simulink model "coursework2model1"  (R2024b)
settings: Solver=VariableStepAuto  StartTime=0.0  StopTime=T  RelTol=1e-3
undefined symbols (not defined in the file): K, x0
settings Model: Creator=user  LastModifiedBy=Oteng_fy0f5z9
settings RTWCC: GPUComputeCapability=3.5

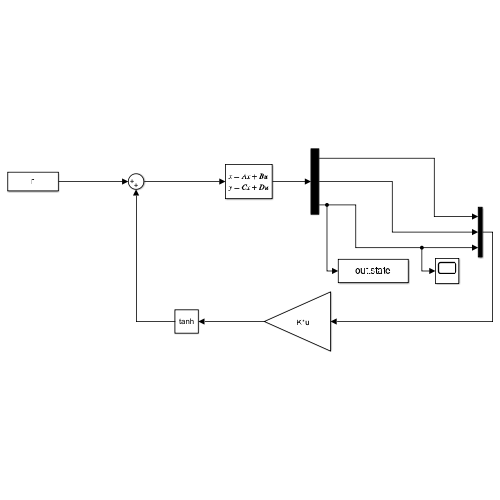
[thumbnail: Simulink's stored preview of the top-level diagram]
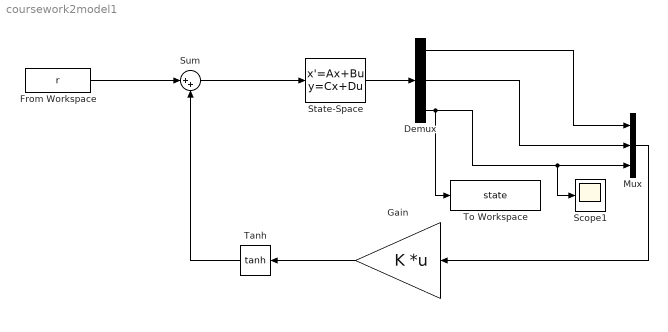
== system coursework2model1 ==
  Demux : Demux  Outputs=3
  From Workspace : FromWorkspace  VariableName=r
  Gain : Gain  Gain=K  Multiplication=Matrix(K*u)
  Mux : Mux  Inputs=3
  Scope1 : Scope
  State-Space : StateSpace  A=[-10 0 10;0 -100 100; 0 0 -1]  B=[0; 0; 1]  C=[1 0 0;0 1 0;0 0 1]  D=[0; 0; 0]  InitialCondition=x0  ParameterTunability=Unconstrained
  Sum : Sum  Inputs=|++
  Tanh : Trigonometry  Operator=tanh
  To Workspace : ToWorkspace  VariableName=state  SaveFormat=Timeseries  SampleTime=-1
  wires:
  Gain/1 -> Tanh/1
  Sum/1 -> State-Space/1
  State-Space/1 -> Demux/1
  Demux/2 -> Mux/2
  Demux/3 -> Scope1/1, Mux/3, To Workspace/1
  Mux/1 -> Gain/1
  Tanh/1 -> Sum/2
  From Workspace/1 -> Sum/1
  Demux/1 -> Mux/1
